simulink model "model1"  (R2024a)
settings: Solver=VariableStepAuto  StartTime=0.0  StopTime=simulation_time  RelTol=1e-3
values from neighbouring files (symbols this model uses):
  dq_0 = zeros(n, 1)    [example.m]
  path = @(t) circle_center + u_circle_plane*radius*cos((t/T) * (2*pi)) + v_circle_plane*radius*sin((t/T) * (2*pi))    [example.m]
  path_ddot = @(t) -u_circle_plane*radius*(2*pi/T)*(2*pi/T)*cos((t/T) * (2*pi)) - v_circle_plane*radius*(2*pi/T)*(2*pi/T)*sin((t/T) * (2*pi))    [example.m]
  path_dot = @(t) -u_circle_plane*radius*(2*pi/T)*sin((t/T) * (2*pi)) + v_circle_plane*radius*(2*pi/T)*cos((t/T) * (2*pi))    [example.m]
  q_0 = randn(n, 1)    [example.m]
  robot_model = importrobot("../robot_model/kuka-lwr-4plus/model1.urdf", 'DataFormat', 'column')    [example.m]
undefined symbols (not defined in the file or in its folder): torque_low_bound, torque_up_bound, X, Y, Z
libraries: sm_lib x74, nesl_utility x8, robotmaniplib x4
(part 5 of 5)

== matlab function model1/MATLAB Function2 ==
  data: configuration input; ee_pos output
% function A0e = get_ee_pos(configuration)
function ee_pos = get_ee_pos(configuration)
%F_Q1
%    OUT1 = F_Q1(Q1,Q2,Q3,Q4)

%    This function was generated by the Symbolic Math Toolbox version 24.1.
%    02-Jul-2024 11:07:49
q1 = configuration(1);
q2 = configuration(2);
q3 = configuration(3);
q4 = configuration(4);

t2 = cos(q1);
t3 = cos(q2);
t4 = cos(q3);
t5 = cos(q4);
t6 = sin(q1);
t7 = sin(q2);
t8 = sin(q3);
t9 = sin(q4);
ee_pos = [t9.*(t6.*t8-t2.*t3.*t4).*(-3.9e+1./1.0e+2)-t2.*t7.*(2.0./5.0)-t2.*t5.*t7.*(3.9e+1./1.0e+2);t9.*(t2.*t8+t3.*t4.*t6).*(3.9e+1./1.0e+2)-t6.*t7.*(2.0./5.0)-t5.*t6.*t7.*(3.9e+1./1.0e+2);t3.*(2.0./5.0)+t3.*t5.*(3.9e+1./1.0e+2)+t4.*t7.*t9.*(3.9e+1./1.0e+2)+3.1e+1./1.0e+2];
end
